simulink model "planta"  (R2014b)
settings: Solver=ode45  StartTime=0.0  StopTime=10.0  RelTol=1e-3
settings Model: Creator=Javi  LastModifiedBy=Javi

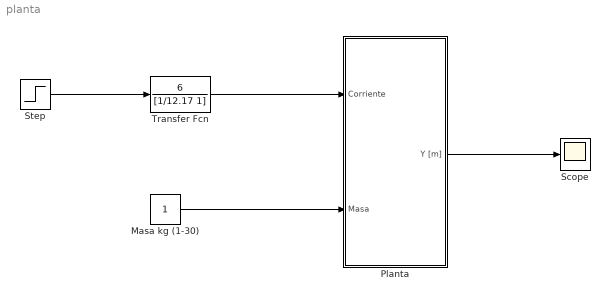
== system planta ==
  Masa kg (1-30) : Constant
  "Planta " : Subsystem
  Scope : Scope
  Step : Step  SampleTime=0
  Transfer Fcn : TransferFcn  Numerator=6  Denominator=[1/12.17 1]
  wires:
  Step/1 -> Transfer Fcn/1
  Transfer Fcn/1 -> "Planta "/1(Corriente)
  Masa kg (1-30)/1 -> "Planta "/2("Masa ")
  "Planta "/1(Y [m]) -> Scope/1

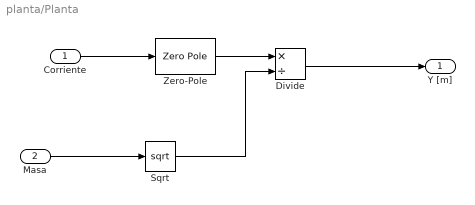
== system planta/Planta  ==
  Corriente : Inport
  "Masa " : Inport  Port=2
  Divide : Product  Inputs=*/
  Sqrt : Sqrt  SaturateOnIntegerOverflow=on
  Zero-Pole : ZeroPole  Zeros=[]  Poles=[70 -70]  Gain=-6.58
  Y [m] : Outport
  wires:
  Divide/1 -> Y [m]/1
  Corriente/1 -> Zero-Pole/1
  Zero-Pole/1 -> Divide/1
  "Masa "/1 -> Sqrt/1
  Sqrt/1 -> Divide/2
